simulink model "satellitsimuppgiftv2"  (R2015a)
settings: Solver=ode45  StartTime=0.0  StopTime=50  RelTol=1e-3
libraries: simulink x4
settings Model: Creator=CTGIKO  LastModifiedBy=Martin
settings DebuggingCC: UnderspecifiedInitializationDetection=Classic  MergeDetectMultiDrivingBlocksExec=none  SolverPrmCheckMsg=warning

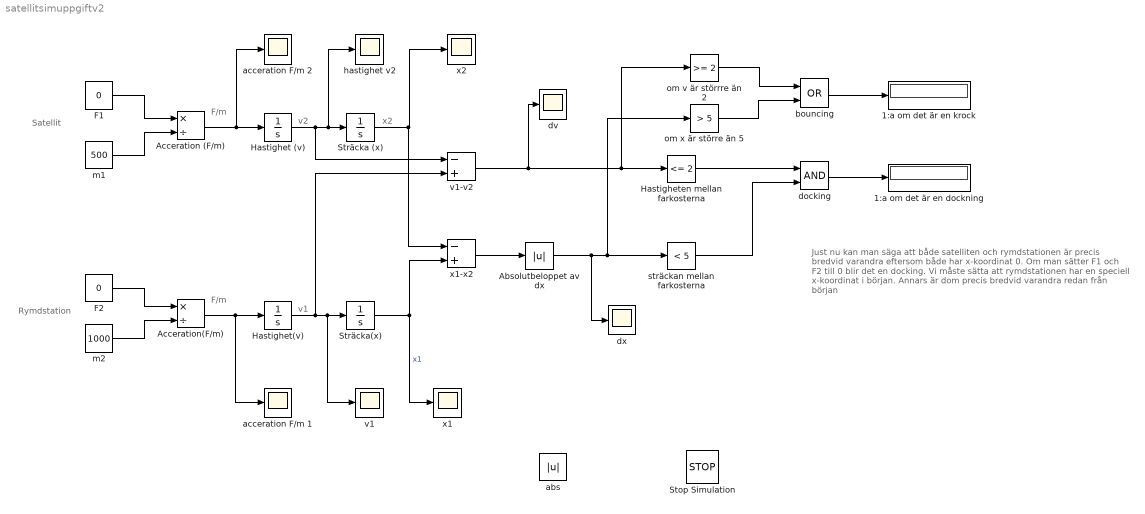
== system satellitsimuppgiftv2 ==
  note: Just nu kan man säga att både satelliten och rymdstationen är precis bredvid varandra eftersom både har x-koordinat 0. Om man sätter F1 och F2 till 0 blir det en docking. Vi måste sätta att rymdstationen har en speciell x-koordinat i början. Annars är dom precis bredvid varandra redan från början
  note: Satellit
  note: Rymdstation
  note: x2
  note: v2
  note: v1
  note: F/m
  note: F/m
  1:a om det är en dockning : Display
  1:a om det är en krock : Display
  Absolutbeloppet av dx : Abs
  Acceration (F/m) : Product  Inputs=*/
  Acceration(F/m) : Product  Inputs=*/
  F1 : Constant  Value=0
  F2 : Constant  Value=0
  Hastighet (v) : Integrator
  "Hastighet(v) " : Integrator
  Hastigheten mellan farkosterna : simulink/Logic and Bit Operations/Compare To Constant  relop=<=  const=2  OutDataTypeStr=boolean
  Stop Simulation : Stop
  Sträcka (x) : Integrator
  Sträcka(x) : Integrator
  abs : Abs
  acceration F/m 1 : Scope
      settings: YMin=-1  YMax=1  SaveName=ScopeData7
  "acceration F/m 2 " : Scope
      settings: YMin=0.6  YMax=1  SaveName=ScopeData5
  bouncing : Logic  Operator=OR  AllPortsSameDT=off  OutDataTypeStr=boolean
  docking : Logic  AllPortsSameDT=off  OutDataTypeStr=boolean
  dv : Scope
      settings: YMin=0  YMax=3  SaveName=ScopeData4
  dx : Scope
      settings: YMin=0  YMax=70  SaveName=ScopeData2
  "hastighet v2 " : Scope
      settings: TimeRange=50  YMin=0  YMax=25  SaveName=ScopeData6
  m1 : Constant  Value=500
  m2 : Constant  Value=1000
  om v är störrre än 2 : simulink/Logic and Bit Operations/Compare To Constant  relop=>=  const=2  OutDataTypeStr=boolean
  om x är större än 5 : simulink/Logic and Bit Operations/Compare To Constant  relop=>  const=5  OutDataTypeStr=boolean
  sträckan mellan farkosterna : simulink/Logic and Bit Operations/Compare To Constant  relop=<  const=5  OutDataTypeStr=boolean
  v1 : Scope
      settings: YMin=0  YMax=9  SaveName=ScopeData3
  v1-v2 : Sum  Inputs=-+
  x1 : Scope
      settings: YMin=-1  YMax=1
  x1-x2 : Sum  RequirementInfo="{}  %GIDa_15f05e76_4de0_4f12_a2c2_6047e8a824a9"  Inputs=-+
  x2 : Scope
      settings: YMin=0  YMax=0.5
  wires:
  F1/1 -> Acceration (F/m)/1
  m1/1 -> Acceration (F/m)/2
  Acceration (F/m)/1 -> "acceration F/m 2 "/1, Hastighet (v)/1
  m2/1 -> Acceration(F/m)/2
  F2/1 -> Acceration(F/m)/1
  Hastighet (v)/1 -> v1-v2/1, "hastighet v2 "/1, Sträcka (x)/1
  "Hastighet(v) "/1 -> v1-v2/2, v1/1, Sträcka(x)/1
  Acceration(F/m)/1 -> acceration F/m 1/1, "Hastighet(v) "/1
  Sträcka (x)/1 -> x1-x2/1, x2/1
  Sträcka(x)/1 -> x1-x2/2, x1/1  "x1"
  sträckan mellan farkosterna/1 -> docking/2
  Hastigheten mellan farkosterna/1 -> docking/1
  om v är störrre än 2/1 -> bouncing/1
  docking/1 -> 1:a om det är en dockning/1
  bouncing/1 -> 1:a om det är en krock/1
  x1-x2/1 -> Absolutbeloppet av dx/1
  v1-v2/1 -> dv/1, om v är störrre än 2/1, Hastigheten mellan farkosterna/1
  Absolutbeloppet av dx/1 -> dx/1, om x är större än 5/1, sträckan mellan farkosterna/1
  om x är större än 5/1 -> bouncing/2
